simulink model "OL_cruise_pitch"  (R2021a)
settings: Solver=VariableStepAuto  StartTime=0.0  StopTime=30  RelTol=1e-12
values from neighbouring files (symbols this model uses):
  C1 = N*Kd + Kp    (= 1.88646026293)    [lead_lag_comp_def.m]
  C2 = N*Kp    (= 1.88648445063e-07)    [lead_lag_comp_def.m]
  C3 = 1    [lead_lag_comp_def.m]
  C4 = N    (= 148.271702233)    [lead_lag_comp_def.m]
settings Model: Creator=12646  LastModifiedBy=12646

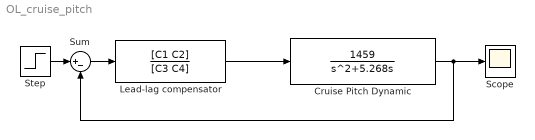
== system OL_cruise_pitch ==
  Cruise Pitch Dynamic : TransferFcn  Numerator=1459  Denominator=[1 5.268 0]
  Lead-lag compensator : TransferFcn  Numerator=[C1 C2]  Denominator=[C3 C4]
  Scope : Scope
  Step : Step  Time=10  SampleTime=0
  Sum : Sum  Inputs=|+-
  wires:
  Lead-lag compensator/1 -> Cruise Pitch Dynamic/1
  Step/1 -> Sum/1
  Cruise Pitch Dynamic/1 -> Sum/2, Scope/1
  Sum/1 -> Lead-lag compensator/1
